simulink model "State"  (R2022b)
settings: Solver=FixedStepAuto  StartTime=0.0  StopTime=10.0  RelTol=1e-3  SampleTimeConstraint=STIndependent
undefined symbols (not defined in the file): C1_Matrix, C2_Matrix, C3_Matrix, Capacity_Vec, Current_Vec, NumberSt, NumModules, NumSeries, R1_Matrix, R2_Matrix, R3_Matrix, RC_SOC_Vec, SOC_Max, SOC_Min, Temperature_Vec, Ts, V1_Max, V1_Min, V2_Max, V2_Min, V3_Max, V3_Min
settings Model: DataDictionary=Estimators_Dictionary.sldd  Creator=japerez  LastModifiedBy=jgavidia
settings DataIOCC: SaveOutput=off  SaveTime=off
settings DebuggingCC: ParameterPrecisionLossMsg=none

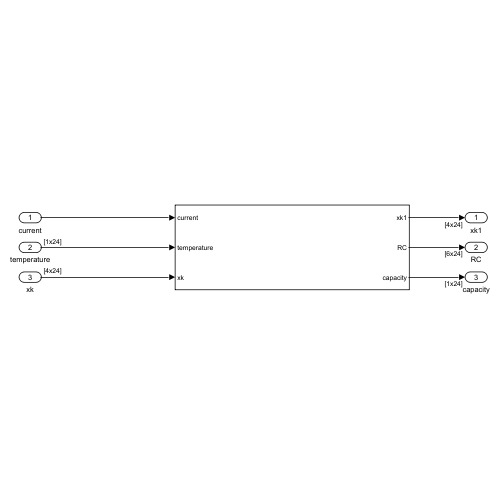
[thumbnail: Simulink's stored preview of the top-level diagram]
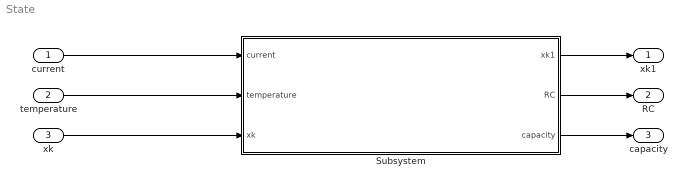
== system State ==
  current : Inport  OutDataTypeStr=single  PortDimensions=1
  temperature : Inport  Port=2  OutDataTypeStr=single  PortDimensions=[1,NumSeries*NumModules]
  xk : Inport  Port=3  OutDataTypeStr=single  PortDimensions=[NumberSt,NumSeries*NumModules]
  Subsystem : Subsystem
  xk1 : Outport  OutDataTypeStr=single  PortDimensions=[NumberSt,NumSeries*NumModules]
  RC : Outport  Port=2  OutDataTypeStr=single  PortDimensions=[6,NumModules*NumSeries]
  capacity : Outport  Port=3  OutDataTypeStr=single  PortDimensions=[1,NumModules*NumSeries]
  wires:
  Subsystem/1(xk1) -> xk1/1
  temperature/1 -> Subsystem/2(temperature)
  Subsystem/2(RC) -> RC/1
  xk/1 -> Subsystem/3(xk)
  Subsystem/3(capacity) -> capacity/1
  current/1 -> Subsystem/1(current)

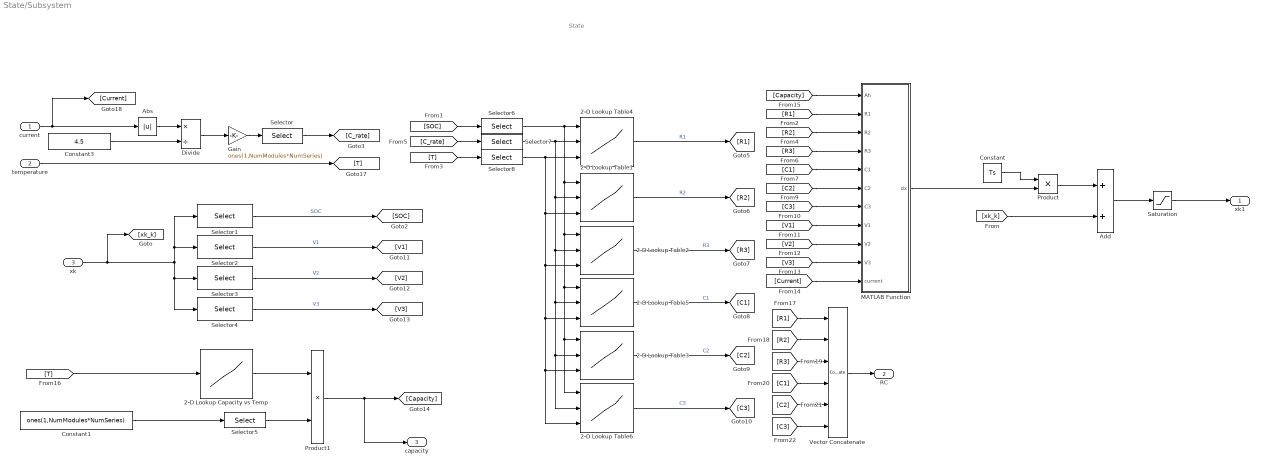
== system State/Subsystem ==
  note: State
  current : Inport
  temperature : Inport  Port=2
  xk : Inport  Port=3
  2-D Lookup Capacity vs Temp : Lookup_n-D  NumberOfTableDimensions=1  BreakpointsForDimension1=Temperature_Vec  BreakpointsForDimension2=Current_Vec  BreakpointsForDimension3=Temperature_Vec  BreakpointsForDimension4=SOH_Vec  Table=Capacity_Vec  InternalRulePriority=Speed  RndMeth=Simplest
  2-D Lookup Table1 : Lookup_n-D  NumberOfTableDimensions=3  BreakpointsForDimension1=RC_SOC_Vec  BreakpointsForDimension2=Current_Vec  BreakpointsForDimension3=Temperature_Vec  BreakpointsForDimension4=SOH_Vec  Table=R2_Matrix  ExtrapMethod=Clip  InternalRulePriority=Speed  RndMeth=Simplest
      settings: InputPortMap=u0,u1,u2
  2-D Lookup Table2 : Lookup_n-D  NumberOfTableDimensions=3  BreakpointsForDimension1=RC_SOC_Vec  BreakpointsForDimension2=Current_Vec  BreakpointsForDimension3=Temperature_Vec  BreakpointsForDimension4=SOH_Vec  Table=R3_Matrix  ExtrapMethod=Clip  InternalRulePriority=Speed  RndMeth=Simplest
      settings: InputPortMap=u0,u1,u2
  2-D Lookup Table3 : Lookup_n-D  NumberOfTableDimensions=3  BreakpointsForDimension1=RC_SOC_Vec  BreakpointsForDimension2=Current_Vec  BreakpointsForDimension3=Temperature_Vec  BreakpointsForDimension4=SOH_Vec  Table=C2_Matrix  ExtrapMethod=Clip  InternalRulePriority=Speed  RndMeth=Simplest
      settings: InputPortMap=u0,u1,u2
  2-D Lookup Table4 : Lookup_n-D  NumberOfTableDimensions=3  BreakpointsForDimension1=RC_SOC_Vec  BreakpointsForDimension2=Current_Vec  BreakpointsForDimension3=Temperature_Vec  BreakpointsForDimension4=SOH_Vec  Table=R1_Matrix  ExtrapMethod=Clip  InternalRulePriority=Speed  RndMeth=Simplest
      settings: InputPortMap=u0,u1,u2
  2-D Lookup Table5 : Lookup_n-D  NumberOfTableDimensions=3  BreakpointsForDimension1=RC_SOC_Vec  BreakpointsForDimension2=Current_Vec  BreakpointsForDimension3=Temperature_Vec  BreakpointsForDimension4=SOH_Vec  Table=C1_Matrix  ExtrapMethod=Clip  InternalRulePriority=Speed  RndMeth=Simplest
      settings: InputPortMap=u0,u1,u2
  2-D Lookup Table6 : Lookup_n-D  NumberOfTableDimensions=3  BreakpointsForDimension1=RC_SOC_Vec  BreakpointsForDimension2=Current_Vec  BreakpointsForDimension3=Temperature_Vec  BreakpointsForDimension4=SOH_Vec  Table=C3_Matrix  ExtrapMethod=Clip  InternalRulePriority=Speed  RndMeth=Simplest
      settings: InputPortMap=u0,u1,u2
  Abs : Abs  SaturateOnIntegerOverflow=off
  Add : Sum  AccumDataTypeStr=single  OutDataTypeStr=single
  Constant : Constant  Value=Ts
  Constant1 : Constant  Value=ones(1,NumModules*NumSeries)  OutDataTypeStr=single
  Constant3 : Constant  Value=4.5  OutDataTypeStr=single
  Divide : Product  Inputs=*/  OutDataTypeStr=single
  Gain : Gain  Gain=ones(1,NumModules*NumSeries)  ParamDataTypeStr=single  OutDataTypeStr=single
  MATLAB Function : MATLAB Function  TreatAsAtomicUnit=on
  Product : Product
  Product1 : Product  OutDataTypeStr=single
  Saturation : Saturate  UpperLimit=[SOC_Max;V1_Max;V2_Max;V3_Max].*ones(NumberSt ,NumModules*NumSeries)  LowerLimit=[SOC_Min;V1_Min;V2_Min;V3_Min].*ones(NumberSt ,NumModules*NumSeries)  OutDataTypeStr=single
  Selector{,5..8} (5 alike) : Selector  NumberOfDimensions=2  InputPortWidth=3  IndexOptions=Select all,Index vector (dialog)  Indices=[1 3],[1:24]  OutputSizes=1,1
  Selector1 : Selector  NumberOfDimensions=2  InputPortWidth=24  IndexOptions=Index vector (dialog),Select all  Indices=1,1  OutputSizes=1,1
  Selector2 : Selector  NumberOfDimensions=2  InputPortWidth=24  IndexOptions=Index vector (dialog),Select all  Indices=2,2  OutputSizes=1,1
  Selector3 : Selector  NumberOfDimensions=2  InputPortWidth=24  IndexOptions=Index vector (dialog),Select all  Indices=3,3  OutputSizes=1,1
  Selector4 : Selector  NumberOfDimensions=2  InputPortWidth=24  IndexOptions=Index vector (dialog),Select all  Indices=4,4  OutputSizes=1,1
  Vector Concatenate : Concatenate  NumInputs=6  Mode=Multidimensional array
  xk1 : Outport
  RC : Outport  Port=2
  capacity : Outport  Port=3
  wires:
  Saturation/1 -> xk1/1
  2-D Lookup Table1/1 -> [R2]  "R2"
  2-D Lookup Capacity vs Temp/1 -> Product1/1
  [R1] -> Vector Concatenate/1
  Vector Concatenate/1 -> RC/1
  Selector1/1 -> [SOC]  "SOC"
  [C2] -> MATLAB Function/6(C2)
  Constant3/1 -> Divide/2
  [V1] -> MATLAB Function/8(V1)
  Product/1 -> Add/1
  MATLAB Function/1(dx) -> Product/2
  [Current] -> MATLAB Function/11(current)
  Selector4/1 -> [V3]  "V3"
  [R2] -> MATLAB Function/3(R2)
  Selector3/1 -> [V2]  "V2"
  Constant/1 -> Product/1
  [xk_k] -> Add/2
  2-D Lookup Table3/1 -> [C2]  "C2"
  Constant1/1 -> Selector5/1
  [V2] -> MATLAB Function/9(V2)
  Divide/1 -> Gain/1
  temperature/1 -> [T]
  [Capacity] -> MATLAB Function/1(Ah)
  [R2] -> Vector Concatenate/2
  Add/1 -> Saturation/1
  [C2] -> Vector Concatenate/5
  [R3] -> Vector Concatenate/3
  2-D Lookup Table5/1 -> [C1]  "C1"
  Abs/1 -> Divide/1
  2-D Lookup Table6/1 -> [C3]  "C3"
  2-D Lookup Table4/1 -> [R1]  "R1"
  2-D Lookup Table2/1 -> [R3]  "R3"
  Selector2/1 -> [V1]  "V1"
  [C_rate] -> Selector7/1
  [C3] -> MATLAB Function/7(C3)
  Product1/1 -> [Capacity], capacity/1
  [T] -> Selector8/1
  [SOC] -> Selector6/1
  xk/1 -> [xk_k], Selector1/1, Selector2/1, Selector4/1, Selector3/1
  [V3] -> MATLAB Function/10(V3)
  [C1] -> MATLAB Function/5(C1)
  [C1] -> Vector Concatenate/4
  [C3] -> Vector Concatenate/6
  [R1] -> MATLAB Function/2(R1)
  current/1 -> [Current], Abs/1
  Gain/1 -> Selector/1
  [R3] -> MATLAB Function/4(R3)
  [T] -> 2-D Lookup Capacity vs Temp/1
  Selector/1 -> [C_rate]
  Selector5/1 -> Product1/2
  Selector6/1 -> 2-D Lookup Table4/1, 2-D Lookup Table3/1, 2-D Lookup Table6/1, 2-D Lookup Table5/1, 2-D Lookup Table2/1, 2-D Lookup Table1/1
  Selector7/1 -> 2-D Lookup Table4/2, 2-D Lookup Table3/2, 2-D Lookup Table6/2, 2-D Lookup Table5/2, 2-D Lookup Table2/2, 2-D Lookup Table1/2
  Selector8/1 -> 2-D Lookup Table4/3, 2-D Lookup Table3/3, 2-D Lookup Table6/3, 2-D Lookup Table5/3, 2-D Lookup Table2/3, 2-D Lookup Table1/3

== matlab function State/Subsystem/MATLAB Function ==
  data: Ah input; dx output; R1 input; R2 input; R3 input; C1 input; C2 input; C3 input; V1 input; V2 input; V3 input; current input
function dx = fcn(Ah,R1,R2,R3,C1,C2,C3,V1,V2,V3,current)
l=length(R1);
dx = single(zeros(4,l));
% Cq is the battery capacity
dx(1,:) = -1./(Ah*3600)*current;
dx(2,:) = (1./C1)*current-V1./(R1.*C1);
dx(3,:) = (1./C2)*current-V2./(R2.*C2);
dx(4,:) = (1./C3)*current-V3./(R3.*C3);
